simulink model "p01"  (R2016a)
settings: Solver=VariableStepAuto  StartTime=0.0  StopTime=20  RelTol=1e-3
undefined symbols (not defined in the file or in its folder): sigbuilder_block
settings Model: Creator=YYJ-PC  LastModifiedBy=YYJ-PC

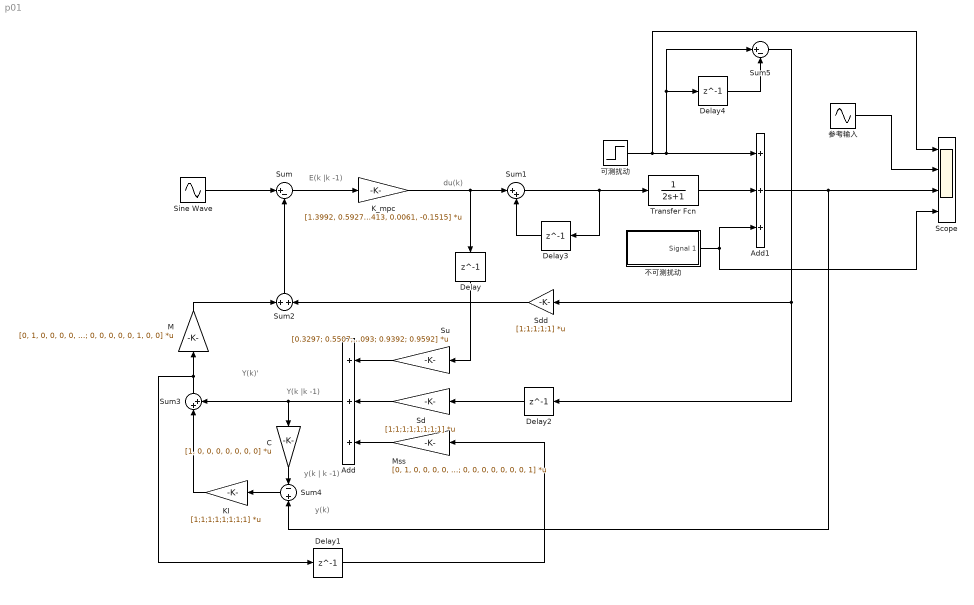
== system p01 ==
  note: du(k)
  note: E(k |k -1)
  note: Y(k)'
  note: Y(k |k -1)
  note: y(k | k -1)
  note: y(k)
  Add : Sum  Inputs=3
  Add1 : Sum  Inputs=3
  C : Gain  Gain=[1, 0, 0, 0, 0, 0, 0, 0]  Multiplication=Matrix(K*u)
  Delay{,1..4} (5 alike) : Delay  DelayLength=1  InitialCondition=0  SampleTime=0.2
  KI : Gain  Gain=[1;1;1;1;1;1;1;1]  Multiplication=Matrix(K*u)
  K_mpc : Gain  Gain=[1.3992, 0.5927, 0.2413, 0.0061, -0.1515]  Multiplication=Matrix(K*u)
  M : Gain  Gain=[0, 1, 0, 0, 0, 0, 0, 0; 0, 0, 1, 0, 0, 0, 0, 0; 0, 0, 0, 1, 0, 0, 0, 0; 0, 0, 0, 0, 1, 0, 0, 0; 0, 0, 0, 0, 0, 1, 0, 0]  Multiplication=Matrix(K*u)
  Mss : Gain  Gain=[0, 1, 0, 0, 0, 0, 0, 0; 0, 0, 1, 0, 0, 0, 0, 0; 0, 0, 0, 1, 0, 0, 0, 0; 0, 0, 0, 0, 1, 0, 0, 0; 0, 0, 0, 0, 0, 1, 0, 0; 0, 0, 0, 0, 0, 0, 1, 0; 0, 0, 0, 0, 0, 0, 0, 1; 0, 0, 0, 0, 0, 0, 0, 1]  Multiplication=Matrix(K*u)
  Scope : Scope  NumInputPorts=4
  "Sd " : Gain  Gain=[1;1;1;1;1;1;1;1]  Multiplication=Matrix(K*u)
  Sdd : Gain  Gain=[1;1;1;1;1]  Multiplication=Matrix(K*u)
  Sine Wave : Sin  Amplitude=2  SampleTime=0.2
  Su : Gain  Gain=|  Multiplication=Matrix(K*u)
      | [0.3297;
      | 0.5507;
      | 0.6988;
      | 0.7981;
      | 0.8647;
      | 0.9093; 0.9392; 0.9592]
  Sum : Sum  Inputs=|+-
  Sum1 : Sum  Inputs=|++
  Sum2 : Sum  Inputs=+|+
  Sum3 : Sum  Inputs=|++
  Sum4 : Sum  Inputs=-|+
  Sum5 : Sum  Inputs=|+-
  Transfer Fcn : TransferFcn  Denominator=[2 1]
  不可测扰动 : Subsystem  Tag=STV Subsys  LoadFcn=sigbuilder_block('load');  StartFcn=sigbuilder_block('start');  StopFcn=sigbuilder_block('stop');  ClipboardFcn=sigbuilder_block('clipboard');  mask(Sigbuilder block){}
      mask help: Simulink:masks:SigbuilderBlock_MD
      mask init:
      | if ~strcmp(get_param(bdroot(gcbh),'SimulationStatus'),'stopped') tuvar = sigbuilder_block('maskInit'); end
      settings: CopyFcn=sigbuilder_block('copy');  DeleteFcn=sigbuilder_block('delete');  ModelCloseFcn=sigbuilder_block('modelClose');  PreSaveFcn=sigbuilder_block('preSave');  PauseFcn=sigbuilder_block('pause');  ContinueFcn=sigbuilder_block('continue');  NameChangeFcn=sigbuilder_block('namechange');  OpenFcn=sigbuilder_block('open',[437.6 199.2 550.4 400 ]);  CloseFcn=sigbuilder_block('close');
      mask Display: plot(0, 0, 100, 100,[2, 2, 32, 32, 2], [68, 8, 8, 68, 68],[32, 2], [38, 38], [32, 19, 2],[53, 60, 44], [32, 17, 17, 2],[16, 16, 31, 31]);txt = getActiveGroup(gcbh);text(2, 100, txt,'verticalAlignment', 'top');
  参考输入 : Sin  Amplitude=2  SampleTime=0
  可测扰动 : Step  SampleTime=0.2
  wires:
  K_mpc/1 -> Delay/1, Sum1/1
  Sum2/1 -> Sum/2
  Su/1 -> Add/1
  Mss/1 -> Add/3
  Sine Wave/1 -> Sum/1
  Sum/1 -> K_mpc/1
  M/1 -> Sum2/1
  Sum3/1 -> M/1, Delay1/1
  C/1 -> Sum4/1
  Sum4/1 -> KI/1
  Delay/1 -> Su/1
  KI/1 -> Sum3/1
  Delay1/1 -> Mss/1
  Delay2/1 -> "Sd "/1
  Delay3/1 -> Sum1/2
  Sum1/1 -> Transfer Fcn/1, Delay3/1
  Sdd/1 -> Sum2/2
  Transfer Fcn/1 -> Add1/2
  可测扰动/1 -> Scope/1, Add1/1, Delay4/1, Sum5/1
  Delay4/1 -> Sum5/2
  Sum5/1 -> Delay2/1, Sdd/1
  "Sd "/1 -> Add/2
  Add/1 -> Sum3/2, C/1
  Add1/1 -> Scope/3, Sum4/2
  不可测扰动/1(Signal 1) -> Scope/4, Add1/3
  参考输入/1 -> Scope/2

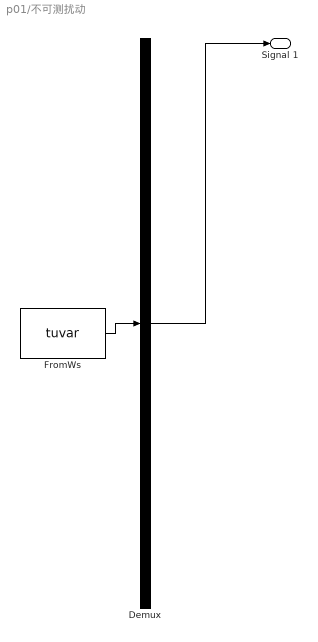
== system p01/不可测扰动 ==
  Demux : Demux  Tag=STV Demux  Outputs=1
  FromWs : FromWorkspace  Tag=STV FromWs  VariableName=tuvar  SampleTime=0
      SigBuilderData=|
      | common.afterFinalStr = 'Extrapolate'
      | common.sampleTime = 0
      | dataSet.timeRange = [0 10]
      | dataSet.name = 'Group 1'
      | sbobj.Groups.Name = 'Group 1'
      | sbobj.Groups.Signals.Name = 'Signal 1'
      | sbobj.Groups.Signals.XData = [0 3.98 3.98 9.7 9.7 10]
      | sbobj.Groups.Signals.YData = [0 0 0.59 0.595 0 0]
  Signal 1 : Outport  Tag=STV Outport
  wires:
  Demux/1 -> Signal 1/1
  FromWs/1 -> Demux/1
